simulink model "gen_smc_quadcopter"  (Simulink 7.9)
settings: Solver=ode4  StartTime=0.0  StopTime=t_end  FixedStep=.001  RelTol=1e-3
values from neighbouring files (symbols this model uses):
  C = [0 0 0]    [gen_smc_starter.m]    (also in pid_starter.m; sliding_starter.m)
  C_nom = [1 1 1].*C    [gen_smc_starter.m]    (also in sliding_starter.m)
  Cd = [0 0 0]    [gen_smc_starter.m]    (also in pid_starter.m; sliding_starter.m)
  Cd_nom = [1 1 1].*Cd    [gen_smc_starter.m]    (also in sliding_starter.m)
  eta = [1 1 1 1]'    [gen_smc_starter.m]    (also in sliding_starter.m = [1 1 1 1 1 1]')
  g = 9.81    [gen_smc_starter.m]    (also in pid_starter.m; sliding_starter.m)
  I = [Ix Iy Iz]    [gen_smc_starter.m]    (also in pid_starter.m; sliding_starter.m)
  Ix_nom = Ix    (= 0.00416666666667)    [gen_smc_starter.m]    (also in sliding_starter.m = 0.00104166666667)
  Iy_nom = Iy    (= 0.00416666666667)    [gen_smc_starter.m]    (also in sliding_starter.m = 0.00104166666667)
  Iz_nom = Iz    (= 0.03125)    [gen_smc_starter.m]    (also in sliding_starter.m)
  Kd = .15*[1 1]    [gen_smc_starter.m]    (also in pid_starter.m = [.01 .01 .6 .001 .001 0])
  Kf = 100    [gen_smc_starter.m]    (also in pid_starter.m; sliding_starter.m)
  Km = 1    [gen_smc_starter.m]    (also in pid_starter.m; sliding_starter.m)
  Kp = .2*[1 1]    [gen_smc_starter.m]    (also in pid_starter.m = [.01 .01 1 .035 .035 60])
  l = .25    (= 0.25)    [gen_smc_starter.m]    (also in pid_starter.m; sliding_starter.m)
  lamb = [1 200 1 1]    [gen_smc_starter.m]    (also in sliding_starter.m = [5 100 5 .1 .1 .1])
  m = .5    (= 0.5)    [gen_smc_starter.m]    (also in pid_starter.m; sliding_starter.m)
  m_nom = m    (= 0.5)    [gen_smc_starter.m]    (also in sliding_starter.m)
  PSI = [.01 .0005 .001 .001]'    [gen_smc_starter.m]    (also in sliding_starter.m = [.005 .005 .005 .005 .005 .005]')
  ref = [0 .5 .1 0 0 0]    [gen_smc_starter.m]    (also in pid_starter.m = [.1 -.1 .5 0 0 0]; sliding_starter.m = [0 2 1 0 0 0])
  step_time = [0 0 0]    [gen_smc_starter.m]    (also in pid_starter.m; sliding_starter.m)
  x0 = [0 0        0 0        .1 0        0 0        0 0        0 0        ]    [gen_smc_starter.m]    (also in pid_starter.m; sliding_starter.m)
settings Model: Creator=dwai  LastModifiedBy=dwai
settings DataIOCC: LimitDataPoints=off
settings DebuggingCC: AlgebraicLoopMsg=none

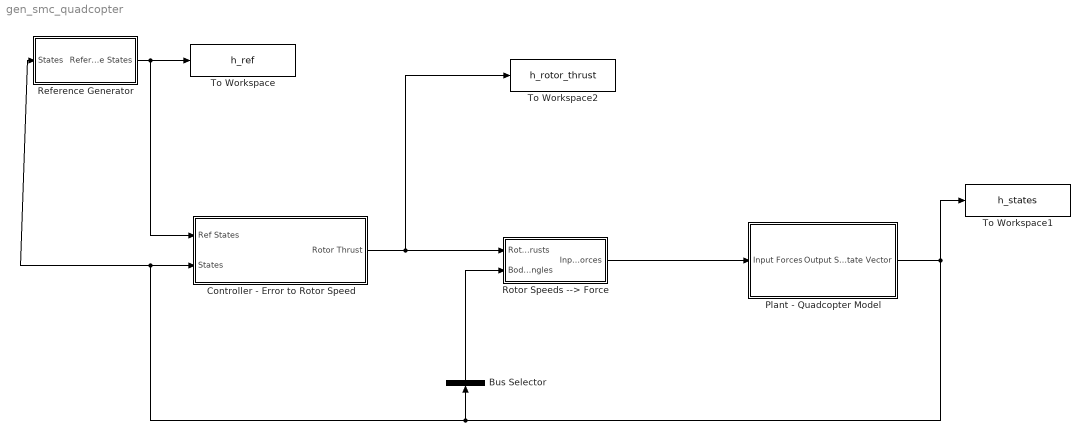
== system gen_smc_quadcopter ==
  Bus Selector : BusSelector  OutputSignals=phi,th,psi  OutputAsBus=on
  Controller - Error to Rotor Speed : Subsystem
  Plant - Quadcopter Model : Subsystem
  Reference Generator : Subsystem
  Rotor Speeds --> Force : Subsystem
  To Workspace : ToWorkspace  VariableName=h_ref  SampleTime=-1  SaveFormat=Timeseries
  To Workspace1 : ToWorkspace  VariableName=h_states  SampleTime=-1  SaveFormat=Timeseries
  To Workspace2 : ToWorkspace  VariableName=h_rotor_thrust  SampleTime=-1  SaveFormat=Timeseries
  wires:
  Plant - Quadcopter Model/1(Output State Vector) -> To Workspace1/1, Bus Selector/1, Controller - Error to Rotor Speed/2(States), Reference Generator/1(States)
  Reference Generator/1(Reference States) -> To Workspace/1, Controller - Error to Rotor Speed/1(Ref States)
  Controller - Error to Rotor Speed/1(Rotor Thrust) -> Rotor Speeds --> Force/1(Rotor Thrusts), To Workspace2/1
  Rotor Speeds --> Force/1(Input Forces) -> Plant - Quadcopter Model/1(Input Forces)
  Bus Selector/1 -> Rotor Speeds --> Force/2(Body Angles)

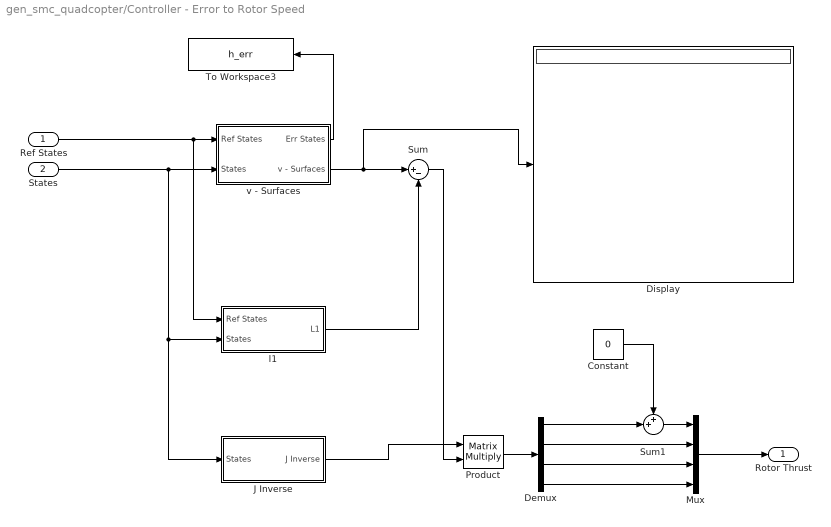
== system gen_smc_quadcopter/Controller - Error to Rotor Speed ==
  Ref States : Inport
  States : Inport  Port=2  PortDimensions=[18 1]
  Constant : Constant  Value=0
  Demux : Demux
  Display : Display
  J Inverse : Subsystem
  Mux : Mux
  Product : Product  Multiplication=Matrix(*)  RndMeth=Zero
  Sum : Sum  Inputs=|+-
  Sum1 : Sum  Inputs=++|
  To Workspace3 : ToWorkspace  VariableName=h_err  SampleTime=-1  SaveFormat=Timeseries
  l1 : Subsystem
  v - Surfaces : Subsystem
  Rotor Thrust : Outport
  wires:
  v - Surfaces/1(Err States) -> To Workspace3/1
  Ref States/1 -> v - Surfaces/1(Ref States), l1/1(Ref States)
  States/1 -> v - Surfaces/2(States), l1/2(States), J Inverse/1(States)
  v - Surfaces/2(v - Surfaces) -> Sum/1, Display/1
  l1/1(L1) -> Sum/2
  J Inverse/1(J Inverse) -> Product/1
  Sum/1 -> Product/2
  Constant/1 -> Sum1/1
  Product/1 -> Demux/1
  Demux/1 -> Sum1/2
  Sum1/1 -> Mux/1
  Demux/2 -> Mux/2
  Demux/3 -> Mux/3
  Demux/4 -> Mux/4
  Mux/1 -> Rotor Thrust/1

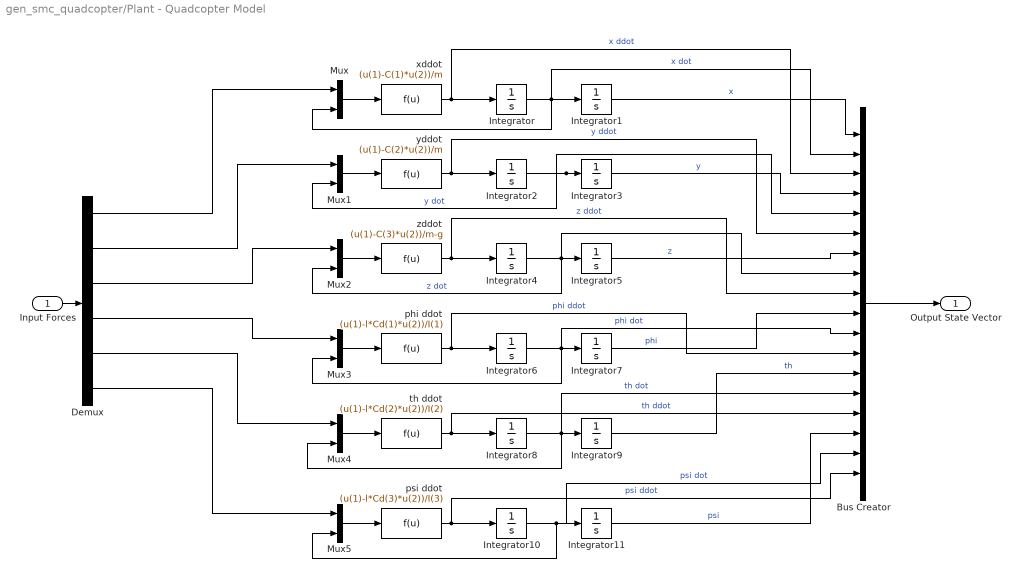
== system gen_smc_quadcopter/Plant - Quadcopter Model ==
  Input Forces : Inport
  Bus Creator : BusCreator  Inputs=18
  Demux : Demux  Outputs=6
  Integrator : Integrator  InitialCondition=x0(2)
  Integrator1 : Integrator  InitialCondition=x0(1)
  Integrator10 : Integrator  InitialCondition=x0(12)
  Integrator11 : Integrator  InitialCondition=x0(11)
  Integrator2 : Integrator  InitialCondition=x0(4)
  Integrator3 : Integrator  InitialCondition=x0(3)
  Integrator4 : Integrator  InitialCondition=x0(6)
  Integrator5 : Integrator  InitialCondition=x0(5)
  Integrator6 : Integrator  InitialCondition=x0(8)
  Integrator7 : Integrator  InitialCondition=x0(7)
  Integrator8 : Integrator  InitialCondition=x0(10)
  Integrator9 : Integrator  InitialCondition=x0(9)
  Mux{,1..5} (6 alike) : Mux  Inputs=2
  phi ddot : Fcn  Expr=(u(1)-l*Cd(1)*u(2))/I(1)
  psi ddot : Fcn  Expr=(u(1)-l*Cd(3)*u(2))/I(3)
  th ddot : Fcn  Expr=(u(1)-l*Cd(2)*u(2))/I(2)
  xddot : Fcn  Expr=(u(1)-C(1)*u(2))/m
  yddot : Fcn  Expr=(u(1)-C(2)*u(2))/m
  zddot : Fcn  Expr=(u(1)-C(3)*u(2))/m-g
  Output State Vector : Outport
  wires:
  Demux/6 -> Mux5/1
  Demux/5 -> Mux4/1
  Demux/4 -> Mux3/1
  Demux/3 -> Mux2/1
  Demux/2 -> Mux1/1
  Demux/1 -> Mux/1
  Integrator11/1 -> Bus Creator/16  "psi"
  Integrator9/1 -> Bus Creator/13  "th"
  Integrator7/1 -> Bus Creator/10  "phi"
  Integrator5/1 -> Bus Creator/7  "z"
  Integrator3/1 -> Bus Creator/4  "y"
  Integrator1/1 -> Bus Creator/1  "x"
  Integrator10/1 -> Integrator11/1, Mux5/2, Bus Creator/17  "psi dot"
  psi ddot/1 -> Integrator10/1, Bus Creator/18  "psi ddot"
  Mux5/1 -> psi ddot/1
  Integrator8/1 -> Integrator9/1, Mux4/2, Bus Creator/14  "th dot"
  th ddot/1 -> Integrator8/1, Bus Creator/15  "th ddot"
  Mux4/1 -> th ddot/1
  Integrator6/1 -> Integrator7/1, Mux3/2, Bus Creator/11  "phi dot"
  phi ddot/1 -> Integrator6/1, Bus Creator/12  "phi ddot"
  Mux3/1 -> phi ddot/1
  Integrator4/1 -> Integrator5/1, Mux2/2, Bus Creator/8  "z dot"
  zddot/1 -> Integrator4/1, Bus Creator/9  "z ddot"
  Mux2/1 -> zddot/1
  Integrator2/1 -> Integrator3/1, Mux1/2, Bus Creator/5  "y dot"
  yddot/1 -> Integrator2/1, Bus Creator/6  "y ddot"
  Mux1/1 -> yddot/1
  Integrator/1 -> Integrator1/1, Mux/2, Bus Creator/2  "x dot"
  xddot/1 -> Integrator/1, Bus Creator/3  "x ddot"
  Mux/1 -> xddot/1
  Bus Creator/1 -> Output State Vector/1
  Input Forces/1 -> Demux/1

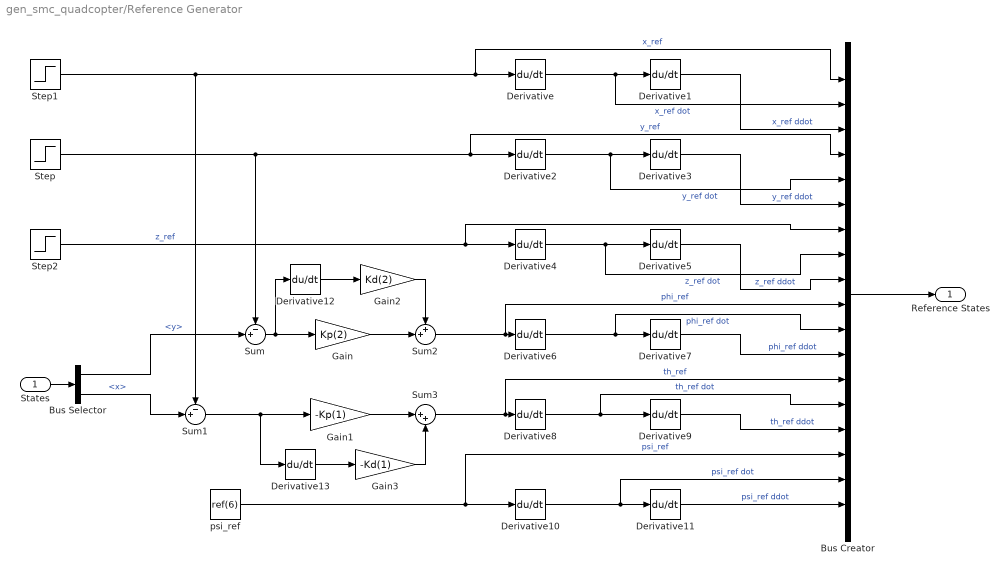
== system gen_smc_quadcopter/Reference Generator ==
  States : Inport
  Bus Creator : BusCreator  Inputs=18
  Bus Selector : BusSelector  OutputSignals=y,x
  Derivative{,1..13} (14 alike) : Derivative
  Gain : Gain  Gain=Kp(2)
  Gain1 : Gain  Gain=-Kp(1)
  Gain2 : Gain  Gain=Kd(2)
  Gain3 : Gain  Gain=-Kd(1)
  Step : Step  Time=step_time(2)  After=ref(2)  SampleTime=0
  Step1 : Step  Time=step_time(1)  After=ref(1)  SampleTime=0
  Step2 : Step  Time=step_time(3)  After=ref(3)  SampleTime=0
  Sum : Sum  Inputs=-+|
  Sum1 : Sum  Inputs=-+|
  Sum2 : Sum  Inputs=++|
  Sum3 : Sum  Inputs=|++
  psi_ref : Constant  Value=ref(6)
  Reference States : Outport
  wires:
  Derivative/1 -> Derivative1/1, Bus Creator/2  "x_ref dot"
  Derivative2/1 -> Derivative3/1, Bus Creator/5  "y_ref dot"
  Step2/1 -> Derivative4/1, Bus Creator/7  "z_ref"
  Derivative4/1 -> Derivative5/1, Bus Creator/8  "z_ref dot"
  Derivative6/1 -> Derivative7/1, Bus Creator/11  "phi_ref dot"
  Derivative8/1 -> Derivative9/1, Bus Creator/14  "th_ref dot"
  psi_ref/1 -> Derivative10/1, Bus Creator/16  "psi_ref"
  Derivative10/1 -> Derivative11/1, Bus Creator/17  "psi_ref dot"
  Derivative1/1 -> Bus Creator/3  "x_ref ddot"
  Derivative3/1 -> Bus Creator/6  "y_ref ddot"
  Derivative5/1 -> Bus Creator/9  "z_ref ddot"
  Derivative7/1 -> Bus Creator/12  "phi_ref ddot"
  Derivative9/1 -> Bus Creator/15  "th_ref ddot"
  Derivative11/1 -> Bus Creator/18  "psi_ref ddot"
  Bus Creator/1 -> Reference States/1
  Step/1 -> Derivative2/1, Bus Creator/4, Sum/1  "y_ref"
  Step1/1 -> Derivative/1, Bus Creator/1, Sum1/1  "x_ref"
  States/1 -> Bus Selector/1
  Sum1/1 -> Gain1/1, Derivative13/1
  Bus Selector/1 -> Sum/2  "<y>"
  Bus Selector/2 -> Sum1/2  "<x>"
  Sum/1 -> Gain/1, Derivative12/1
  Sum2/1 -> Bus Creator/10, Derivative6/1  "phi_ref"
  Gain/1 -> Sum2/2
  Gain2/1 -> Sum2/1
  Derivative12/1 -> Gain2/1
  Sum3/1 -> Bus Creator/13, Derivative8/1  "th_ref"
  Gain3/1 -> Sum3/2
  Derivative13/1 -> Gain3/1
  Gain1/1 -> Sum3/1

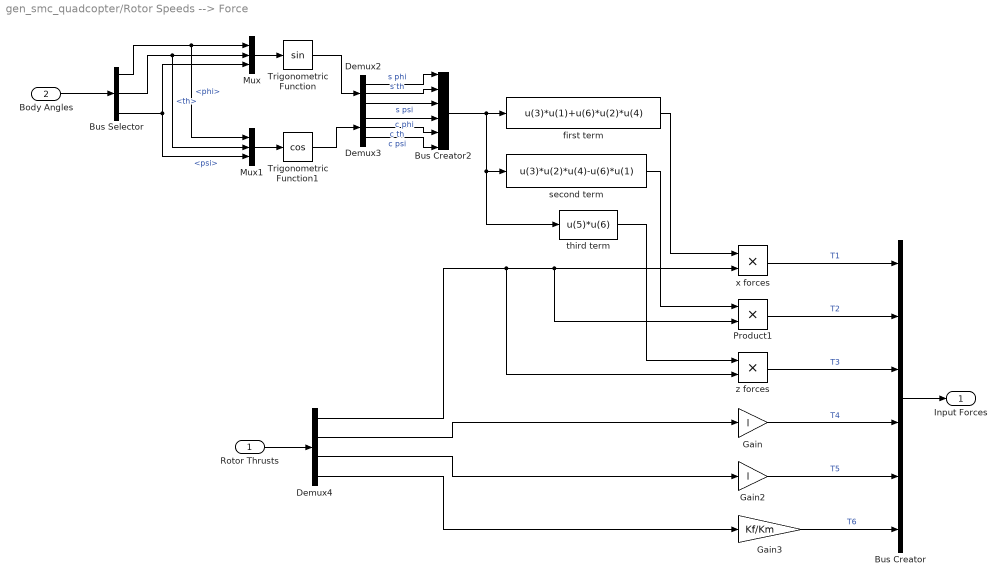
== system gen_smc_quadcopter/Rotor Speeds --> Force ==
  Rotor Thrusts : Inport
  Body Angles : Inport  Port=2
  Bus Creator : BusCreator  Inputs=6
  Bus Creator2 : BusCreator  Inputs=6
  Bus Selector : BusSelector  OutputSignals=phi,th,psi
  Demux2 : Demux  Outputs=3
  Demux3 : Demux  Outputs=3
  Demux4 : Demux
  Gain : Gain  Gain=l
  Gain2 : Gain  Gain=l
  Gain3 : Gain  Gain=Kf/Km
  Mux : Mux  Inputs=3
  Mux1 : Mux  Inputs=3
  Product1 : Product  RndMeth=Zero
  Trigonometric Function : Trigonometry
  Trigonometric Function1 : Trigonometry  Operator=cos
  first term : Fcn  Expr=u(3)*u(1)+u(6)*u(2)*u(4)
  second term : Fcn  Expr=u(3)*u(2)*u(4)-u(6)*u(1)
  third term : Fcn  Expr=u(5)*u(6)
  x forces : Product  RndMeth=Zero
  z forces : Product  RndMeth=Zero
  Input Forces : Outport
  wires:
  Bus Creator/1 -> Input Forces/1
  Body Angles/1 -> Bus Selector/1
  Bus Selector/3 -> Mux/3, Mux1/3  "<psi>"
  Bus Selector/2 -> Mux/2, Mux1/2  "<th>"
  Bus Selector/1 -> Mux/1, Mux1/1  "<phi>"
  Mux/1 -> Trigonometric Function/1
  Mux1/1 -> Trigonometric Function1/1
  Trigonometric Function/1 -> Demux2/1
  Trigonometric Function1/1 -> Demux3/1
  Demux2/1 -> Bus Creator2/1  "s phi"
  Demux2/2 -> Bus Creator2/2  "s th"
  Demux2/3 -> Bus Creator2/3  "s psi"
  Demux3/1 -> Bus Creator2/4  "c phi"
  Demux3/2 -> Bus Creator2/5  "c th"
  Demux3/3 -> Bus Creator2/6  "c psi"
  Bus Creator2/1 -> first term/1, second term/1, third term/1
  x forces/1 -> Bus Creator/1  "T1"
  first term/1 -> x forces/1
  Demux4/1 -> z forces/2, x forces/2, Product1/2
  second term/1 -> Product1/1
  third term/1 -> z forces/1
  Product1/1 -> Bus Creator/2  "T2"
  z forces/1 -> Bus Creator/3  "T3"
  Gain3/1 -> Bus Creator/6  "T6"
  Gain/1 -> Bus Creator/4  "T4"
  Gain2/1 -> Bus Creator/5  "T5"
  Rotor Thrusts/1 -> Demux4/1
  Demux4/2 -> Gain/1
  Demux4/3 -> Gain2/1
  Demux4/4 -> Gain3/1

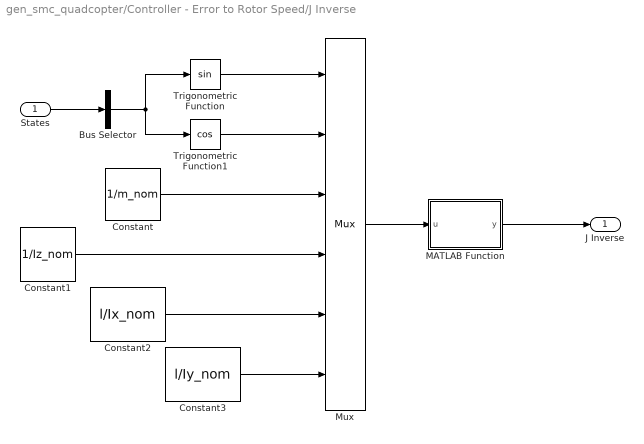
== system gen_smc_quadcopter/Controller - Error to Rotor Speed/J Inverse ==
  States : Inport
  Bus Selector : BusSelector  OutputSignals=phi,th,psi  OutputAsBus=on
  Constant : Constant  Value=1/m_nom
  Constant1 : Constant  Value=1/Iz_nom
  Constant2 : Constant  Value=l/Ix_nom
  Constant3 : Constant  Value=l/Iy_nom
  MATLAB Function : MATLAB Function  TreatAsAtomicUnit=on
  Mux : Mux  Inputs=6
      settings: DisplayOption=signals
  Trigonometric Function : Trigonometry
  Trigonometric Function1 : Trigonometry  Operator=cos
  J Inverse : Outport  PortDimensions=[4 4]
  wires:
  States/1 -> Bus Selector/1
  Bus Selector/1 -> Trigonometric Function/1, Trigonometric Function1/1
  Trigonometric Function1/1 -> Mux/2
  Trigonometric Function/1 -> Mux/1
  Constant/1 -> Mux/3
  Constant1/1 -> Mux/4
  MATLAB Function/1(y) -> J Inverse/1
  Mux/1 -> MATLAB Function/1(u)
  Constant2/1 -> Mux/5
  Constant3/1 -> Mux/6

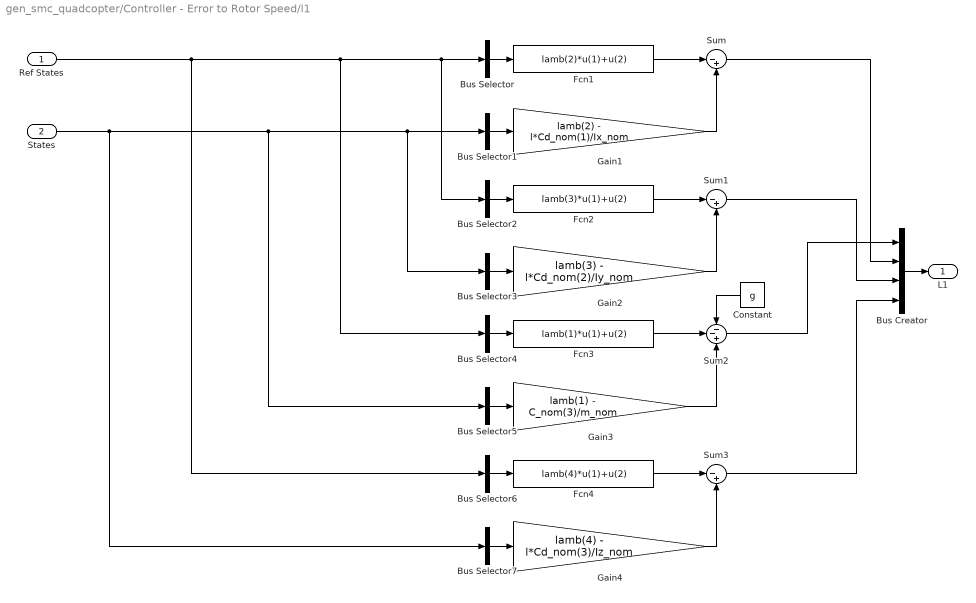
== system gen_smc_quadcopter/Controller - Error to Rotor Speed/l1 ==
  Ref States : Inport
  States : Inport  Port=2
  Bus Creator : BusCreator
  Bus Selector : BusSelector  OutputSignals=phi_ref dot,phi_ref ddot  OutputAsBus=on
  Bus Selector1 : BusSelector  OutputSignals=phi dot  OutputAsBus=on
  Bus Selector2 : BusSelector  OutputSignals=th_ref dot,th_ref ddot  OutputAsBus=on
  Bus Selector3 : BusSelector  OutputSignals=th dot  OutputAsBus=on
  Bus Selector4 : BusSelector  OutputSignals=z_ref dot,z_ref ddot  OutputAsBus=on
  Bus Selector5 : BusSelector  OutputSignals=z dot  OutputAsBus=on
  Bus Selector6 : BusSelector  OutputSignals=psi_ref dot,psi_ref ddot  OutputAsBus=on
  Bus Selector7 : BusSelector  OutputSignals=psi dot  OutputAsBus=on
  Constant : Constant  Value=g
  Fcn1 : Fcn  Expr=lamb(2)*u(1)+u(2)
  Fcn2 : Fcn  Expr=lamb(3)*u(1)+u(2)
  Fcn3 : Fcn  Expr=lamb(1)*u(1)+u(2)
  Fcn4 : Fcn  Expr=lamb(4)*u(1)+u(2)
  Gain1 : Gain  Gain=lamb(2) - l*Cd_nom(1)/Ix_nom
  Gain2 : Gain  Gain=lamb(3) - l*Cd_nom(2)/Iy_nom
  Gain3 : Gain  Gain=lamb(1) - C_nom(3)/m_nom
  Gain4 : Gain  Gain=lamb(4) - l*Cd_nom(3)/Iz_nom
  Sum : Sum  Inputs=|-+
  Sum1 : Sum  Inputs=|-+
  Sum2 : Sum  Inputs=--+
  Sum3 : Sum  Inputs=|-+
  L1 : Outport
  wires:
  Ref States/1 -> Bus Selector/1, Bus Selector2/1, Bus Selector4/1, Bus Selector6/1
  States/1 -> Bus Selector1/1, Bus Selector3/1, Bus Selector5/1, Bus Selector7/1
  Bus Selector1/1 -> Gain1/1
  Bus Selector/1 -> Fcn1/1
  Fcn1/1 -> Sum/1
  Gain1/1 -> Sum/2
  Bus Selector3/1 -> Gain2/1
  Bus Selector2/1 -> Fcn2/1
  Fcn2/1 -> Sum1/1
  Gain2/1 -> Sum1/2
  Bus Selector5/1 -> Gain3/1
  Bus Selector4/1 -> Fcn3/1
  Bus Selector7/1 -> Gain4/1
  Bus Selector6/1 -> Fcn4/1
  Fcn4/1 -> Sum3/1
  Gain4/1 -> Sum3/2
  Constant/1 -> Sum2/1
  Gain3/1 -> Sum2/3
  Fcn3/1 -> Sum2/2
  Bus Creator/1 -> L1/1
  Sum2/1 -> Bus Creator/1
  Sum/1 -> Bus Creator/2
  Sum1/1 -> Bus Creator/3
  Sum3/1 -> Bus Creator/4

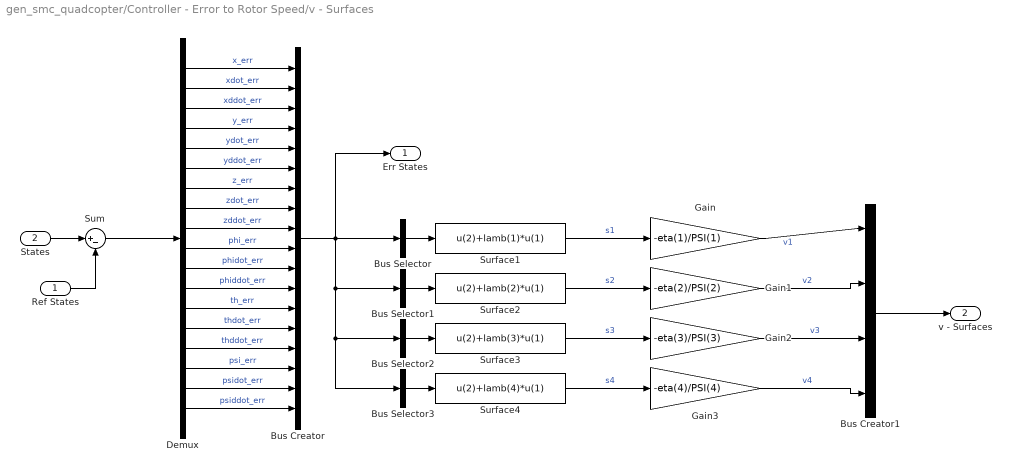
== system gen_smc_quadcopter/Controller - Error to Rotor Speed/v - Surfaces ==
  Ref States : Inport
  States : Inport  Port=2
  Bus Creator : BusCreator  Inputs=18
  Bus Creator1 : BusCreator
  Bus Selector : BusSelector  OutputSignals=z_err,zdot_err  OutputAsBus=on
  Bus Selector1 : BusSelector  OutputSignals=phi_err,phidot_err  OutputAsBus=on
  Bus Selector2 : BusSelector  OutputSignals=th_err,thdot_err  OutputAsBus=on
  Bus Selector3 : BusSelector  OutputSignals=psi_err,psidot_err  OutputAsBus=on
  Demux : Demux  Outputs=18
  Gain : Gain  Gain=-eta(1)/PSI(1)
  Gain1 : Gain  Gain=-eta(2)/PSI(2)
  Gain2 : Gain  Gain=-eta(3)/PSI(3)
  Gain3 : Gain  Gain=-eta(4)/PSI(4)
  Sum : Sum  Inputs=|+-
  Surface1 : Fcn  Expr=u(2)+lamb(1)*u(1)
  Surface2 : Fcn  Expr=u(2)+lamb(2)*u(1)
  Surface3 : Fcn  Expr=u(2)+lamb(3)*u(1)
  Surface4 : Fcn  Expr=u(2)+lamb(4)*u(1)
  Err States : Outport
  v - Surfaces : Outport  Port=2
  wires:
  Bus Creator/1 -> Bus Selector/1, Bus Selector2/1, Bus Selector3/1, Bus Selector1/1, Err States/1
  Demux/18 -> Bus Creator/18  "psiddot_err"
  Demux/17 -> Bus Creator/17  "psidot_err"
  Demux/16 -> Bus Creator/16  "psi_err"
  Demux/15 -> Bus Creator/15  "thddot_err"
  Demux/14 -> Bus Creator/14  "thdot_err"
  Demux/13 -> Bus Creator/13  "th_err"
  Demux/12 -> Bus Creator/12  "phiddot_err"
  Demux/11 -> Bus Creator/11  "phidot_err"
  Demux/10 -> Bus Creator/10  "phi_err"
  Demux/9 -> Bus Creator/9  "zddot_err"
  Demux/8 -> Bus Creator/8  "zdot_err"
  Demux/7 -> Bus Creator/7  "z_err"
  Demux/6 -> Bus Creator/6  "yddot_err"
  Demux/5 -> Bus Creator/5  "ydot_err"
  Demux/4 -> Bus Creator/4  "y_err"
  Demux/3 -> Bus Creator/3  "xddot_err"
  Demux/2 -> Bus Creator/2  "xdot_err"
  Demux/1 -> Bus Creator/1  "x_err"
  Bus Selector/1 -> Surface1/1
  Bus Selector1/1 -> Surface2/1
  Bus Selector2/1 -> Surface3/1
  Bus Selector3/1 -> Surface4/1
  Surface4/1 -> Gain3/1  "s4"
  Surface3/1 -> Gain2/1  "s3"
  Surface2/1 -> Gain1/1  "s2"
  Surface1/1 -> Gain/1  "s1"
  Gain/1 -> Bus Creator1/1  "v1"
  Gain1/1 -> Bus Creator1/2  "v2"
  Gain2/1 -> Bus Creator1/3  "v3"
  Gain3/1 -> Bus Creator1/4  "v4"
  Bus Creator1/1 -> v - Surfaces/1
  States/1 -> Sum/1
  Ref States/1 -> Sum/2
  Sum/1 -> Demux/1

== matlab function Controller - Error to Rotor Speed/J Inverse/MATLAB Function ==
  data: u input double; y output double
function y = fcn(u)

s_phi = u(1);
s_th = u(2);
s_psi = u(3);
c_phi = u(4);
c_th = u(5);
c_psi = u(6);
a = u(7); %1/m
b = u(8); %1/Iz
c = u(9); %l/Ix
d = u(10); %l/Iy
    
J = diag([a*(c_th*c_psi) c d b]);
y = inv(J);
